simulink model "fusionAlg"  (R2018b)
settings: Solver=FixedStepDiscrete  StartTime=0.0  StopTime=inf  FixedStep=0.01  RelTol=1e-3
PostLoadFcn:
  | if any(exist('dsrtsu_mdlpostloadfcn', 'file') ~= 0), dsrtsu_mdlpostloadfcn('Execute', bdroot); end
model workspace (MAT data in the model file):
  handle : class17 (value not decoded)
(part 11 of 24)

== system fusionAlg/FUSION /FusionAlg/BusToBusArray/BusToBusArray/FUS_Obj_30 ==
  <fus_output_30_obj> : Inport
  Bus Creator : BusCreator  Inputs=15  OutDataTypeStr=Bus: FUS_OBJ_TRACK_EST_ST  NonVirtualBus=on
      settings: InheritFromInputs=off
  Bus Creator1 : BusCreator  Inputs=15  OutDataTypeStr=Bus: FUS_OBJ_TRACK_PROP_ST  NonVirtualBus=on
      settings: InheritFromInputs=off
  Bus Creator2 : BusCreator  Inputs=10  OutDataTypeStr=Bus: FUS_OBJ_TRACK_INFO_ST  NonVirtualBus=on
      settings: InheritFromInputs=off
  Bus Creator3 : BusCreator  Inputs=3  OutDataTypeStr=Bus: FUS_OBJ_DATA_ST  NonVirtualBus=on
      settings: InheritFromInputs=off
  Bus Selector : BusSelector  OutputSignals=obj_estimate,obj_property,obj_information
  Bus Selector1 : BusSelector  OutputSignals=longPosition,latPosition,headingAngle,speed,yawRate,longRelativeVelocity,latRelativeVelocity,longAbsoluteVelocity,latAbsoluteVelocity,acceleration,longRelativeAcceleration,latRelativeAcceleration,longAbsoluteAcceleration,latAbsoluteAcceleration,curvature
  Bus Selector2 : BusSelector  OutputSignals=id,fusionSource,motionModel,trackStatus,positionConfidence,fcwConfidence,tjaConfidence,leftNearLaneMarkingConfidence,rightNearLaneMarkingConfidence,visionId,accelerationStdDev,headingAngleStdDev,latPositionStdDev,longPositionStdDev,speedStdDev
  Bus Selector3 : BusSelector  OutputSignals=valid,type,nearestSide,motionPatternCurrent,motionPatternHistory,width,height,length,distanceToleftNearLaneMarking,distanceToRightNearLaneMarking
  BUS_fus_output_30_obj : Outport
  wires:
  <fus_output_30_obj>/1 -> Bus Selector/1
  Bus Selector/1 -> Bus Selector1/1  "<obj_estimate>"
  Bus Selector1/1 -> Bus Creator/1  "<longPosition>"
  Bus Selector1/2 -> Bus Creator/2  "<latPosition>"
  Bus Selector1/4 -> Bus Creator/4  "<speed>"
  Bus Selector1/5 -> Bus Creator/5  "<yawRate>"
  Bus Selector1/6 -> Bus Creator/6  "<longRelativeVelocity>"
  Bus Selector1/3 -> Bus Creator/3  "<headingAngle>"
  Bus Selector1/7 -> Bus Creator/7  "<latRelativeVelocity>"
  Bus Selector/2 -> Bus Selector2/1  "<obj_property>"
  Bus Selector/3 -> Bus Selector3/1  "<obj_information>"
  Bus Selector2/1 -> Bus Creator1/1  "<id>"
  Bus Selector2/2 -> Bus Creator1/2  "<fusionSource>"
  Bus Selector2/3 -> Bus Creator1/3  "<motionModel>"
  Bus Selector2/4 -> Bus Creator1/4  "<trackStatus>"
  Bus Selector2/6 -> Bus Creator1/6  "<fcwConfidence>"
  Bus Selector2/11 -> Bus Creator1/11  "<accelerationStdDev>"
  Bus Selector2/12 -> Bus Creator1/12  "<headingAngleStdDev>"
  Bus Selector2/13 -> Bus Creator1/13  "<latPositionStdDev>"
  Bus Selector2/14 -> Bus Creator1/14  "<longPositionStdDev>"
  Bus Selector2/15 -> Bus Creator1/15  "<speedStdDev>"
  Bus Selector2/9 -> Bus Creator1/9  "<rightNearLaneMarkingConfidence>"
  Bus Selector2/8 -> Bus Creator1/8  "<leftNearLaneMarkingConfidence>"
  Bus Selector2/10 -> Bus Creator1/10  "<visionId>"
  Bus Selector2/5 -> Bus Creator1/5  "<positionConfidence>"
  Bus Selector2/7 -> Bus Creator1/7  "<tjaConfidence>"
  Bus Selector3/1 -> Bus Creator2/1  "<valid>"
  Bus Selector3/2 -> Bus Creator2/2  "<type>"
  Bus Selector3/3 -> Bus Creator2/3  "<nearestSide>"
  Bus Selector3/4 -> Bus Creator2/4  "<motionPatternCurrent>"
  Bus Selector3/5 -> Bus Creator2/5  "<motionPatternHistory>"
  Bus Selector3/6 -> Bus Creator2/6  "<width>"
  Bus Selector3/7 -> Bus Creator2/7  "<height>"
  Bus Selector3/8 -> Bus Creator2/8  "<length>"
  Bus Selector3/9 -> Bus Creator2/9  "<distanceToleftNearLaneMarking>"
  Bus Creator/1 -> Bus Creator3/1
  Bus Creator1/1 -> Bus Creator3/2
  Bus Creator2/1 -> Bus Creator3/3
  Bus Creator3/1 -> BUS_fus_output_30_obj/1
  Bus Selector3/10 -> Bus Creator2/10  "<distanceToRightNearLaneMarking>"
  Bus Selector1/8 -> Bus Creator/8  "<longAbsoluteVelocity>"
  Bus Selector1/9 -> Bus Creator/9  "<latAbsoluteVelocity>"
  Bus Selector1/10 -> Bus Creator/10  "<acceleration>"
  Bus Selector1/11 -> Bus Creator/11  "<longRelativeAcceleration>"
  Bus Selector1/12 -> Bus Creator/12  "<latRelativeAcceleration>"
  Bus Selector1/13 -> Bus Creator/13  "<longAbsoluteAcceleration>"
  Bus Selector1/14 -> Bus Creator/14  "<latAbsoluteAcceleration>"
  Bus Selector1/15 -> Bus Creator/15  "<curvature>"

== system fusionAlg/FUSION /FusionAlg/BusToBusArray/BusToBusArray/FUS_Obj_31 ==
  <fus_output_31_obj> : Inport
  Bus Creator : BusCreator  Inputs=15  OutDataTypeStr=Bus: FUS_OBJ_TRACK_EST_ST  NonVirtualBus=on
      settings: InheritFromInputs=off
  Bus Creator1 : BusCreator  Inputs=15  OutDataTypeStr=Bus: FUS_OBJ_TRACK_PROP_ST  NonVirtualBus=on
      settings: InheritFromInputs=off
  Bus Creator2 : BusCreator  Inputs=10  OutDataTypeStr=Bus: FUS_OBJ_TRACK_INFO_ST  NonVirtualBus=on
      settings: InheritFromInputs=off
  Bus Creator3 : BusCreator  Inputs=3  OutDataTypeStr=Bus: FUS_OBJ_DATA_ST  NonVirtualBus=on
      settings: InheritFromInputs=off
  Bus Selector : BusSelector  OutputSignals=obj_estimate,obj_property,obj_information
  Bus Selector1 : BusSelector  OutputSignals=longPosition,latPosition,headingAngle,speed,yawRate,longRelativeVelocity,latRelativeVelocity,longAbsoluteVelocity,latAbsoluteVelocity,acceleration,longRelativeAcceleration,latRelativeAcceleration,longAbsoluteAcceleration,latAbsoluteAcceleration,curvature
  Bus Selector2 : BusSelector  OutputSignals=id,fusionSource,motionModel,trackStatus,positionConfidence,fcwConfidence,tjaConfidence,leftNearLaneMarkingConfidence,rightNearLaneMarkingConfidence,visionId,accelerationStdDev,headingAngleStdDev,latPositionStdDev,longPositionStdDev,speedStdDev
  Bus Selector3 : BusSelector  OutputSignals=valid,type,nearestSide,motionPatternCurrent,motionPatternHistory,width,height,length,distanceToleftNearLaneMarking,distanceToRightNearLaneMarking
  BUS_fus_output_31_obj : Outport
  wires:
  <fus_output_31_obj>/1 -> Bus Selector/1
  Bus Selector/1 -> Bus Selector1/1  "<obj_estimate>"
  Bus Selector1/1 -> Bus Creator/1  "<longPosition>"
  Bus Selector1/2 -> Bus Creator/2  "<latPosition>"
  Bus Selector1/4 -> Bus Creator/4  "<speed>"
  Bus Selector1/5 -> Bus Creator/5  "<yawRate>"
  Bus Selector1/6 -> Bus Creator/6  "<longRelativeVelocity>"
  Bus Selector1/3 -> Bus Creator/3  "<headingAngle>"
  Bus Selector1/7 -> Bus Creator/7  "<latRelativeVelocity>"
  Bus Selector/2 -> Bus Selector2/1  "<obj_property>"
  Bus Selector/3 -> Bus Selector3/1  "<obj_information>"
  Bus Selector2/1 -> Bus Creator1/1  "<id>"
  Bus Selector2/2 -> Bus Creator1/2  "<fusionSource>"
  Bus Selector2/3 -> Bus Creator1/3  "<motionModel>"
  Bus Selector2/4 -> Bus Creator1/4  "<trackStatus>"
  Bus Selector2/6 -> Bus Creator1/6  "<fcwConfidence>"
  Bus Selector2/11 -> Bus Creator1/11  "<accelerationStdDev>"
  Bus Selector2/12 -> Bus Creator1/12  "<headingAngleStdDev>"
  Bus Selector2/13 -> Bus Creator1/13  "<latPositionStdDev>"
  Bus Selector2/14 -> Bus Creator1/14  "<longPositionStdDev>"
  Bus Selector2/15 -> Bus Creator1/15  "<speedStdDev>"
  Bus Selector2/9 -> Bus Creator1/9  "<rightNearLaneMarkingConfidence>"
  Bus Selector2/8 -> Bus Creator1/8  "<leftNearLaneMarkingConfidence>"
  Bus Selector2/10 -> Bus Creator1/10  "<visionId>"
  Bus Selector2/5 -> Bus Creator1/5  "<positionConfidence>"
  Bus Selector2/7 -> Bus Creator1/7  "<tjaConfidence>"
  Bus Selector3/1 -> Bus Creator2/1  "<valid>"
  Bus Selector3/2 -> Bus Creator2/2  "<type>"
  Bus Selector3/3 -> Bus Creator2/3  "<nearestSide>"
  Bus Selector3/4 -> Bus Creator2/4  "<motionPatternCurrent>"
  Bus Selector3/5 -> Bus Creator2/5  "<motionPatternHistory>"
  Bus Selector3/6 -> Bus Creator2/6  "<width>"
  Bus Selector3/7 -> Bus Creator2/7  "<height>"
  Bus Selector3/8 -> Bus Creator2/8  "<length>"
  Bus Selector3/9 -> Bus Creator2/9  "<distanceToleftNearLaneMarking>"
  Bus Creator/1 -> Bus Creator3/1
  Bus Creator1/1 -> Bus Creator3/2
  Bus Creator2/1 -> Bus Creator3/3
  Bus Creator3/1 -> BUS_fus_output_31_obj/1
  Bus Selector3/10 -> Bus Creator2/10  "<distanceToRightNearLaneMarking>"
  Bus Selector1/8 -> Bus Creator/8  "<longAbsoluteVelocity>"
  Bus Selector1/9 -> Bus Creator/9  "<latAbsoluteVelocity>"
  Bus Selector1/10 -> Bus Creator/10  "<acceleration>"
  Bus Selector1/11 -> Bus Creator/11  "<longRelativeAcceleration>"
  Bus Selector1/12 -> Bus Creator/12  "<latRelativeAcceleration>"
  Bus Selector1/13 -> Bus Creator/13  "<longAbsoluteAcceleration>"
  Bus Selector1/14 -> Bus Creator/14  "<latAbsoluteAcceleration>"
  Bus Selector1/15 -> Bus Creator/15  "<curvature>"

== system fusionAlg/FUSION /FusionAlg/BusToBusArray/BusToBusArray/FUS_Obj_32 ==
  <fus_output_32_obj> : Inport
  Bus Creator : BusCreator  Inputs=15  OutDataTypeStr=Bus: FUS_OBJ_TRACK_EST_ST  NonVirtualBus=on
      settings: InheritFromInputs=off
  Bus Creator1 : BusCreator  Inputs=15  OutDataTypeStr=Bus: FUS_OBJ_TRACK_PROP_ST  NonVirtualBus=on
      settings: InheritFromInputs=off
  Bus Creator2 : BusCreator  Inputs=10  OutDataTypeStr=Bus: FUS_OBJ_TRACK_INFO_ST  NonVirtualBus=on
      settings: InheritFromInputs=off
  Bus Creator3 : BusCreator  Inputs=3  OutDataTypeStr=Bus: FUS_OBJ_DATA_ST  NonVirtualBus=on
      settings: InheritFromInputs=off
  Bus Selector : BusSelector  OutputSignals=obj_estimate,obj_property,obj_information
  Bus Selector1 : BusSelector  OutputSignals=longPosition,latPosition,headingAngle,speed,yawRate,longRelativeVelocity,latRelativeVelocity,longAbsoluteVelocity,latAbsoluteVelocity,acceleration,longRelativeAcceleration,latRelativeAcceleration,longAbsoluteAcceleration,latAbsoluteAcceleration,curvature
  Bus Selector2 : BusSelector  OutputSignals=id,fusionSource,motionModel,trackStatus,positionConfidence,fcwConfidence,tjaConfidence,leftNearLaneMarkingConfidence,rightNearLaneMarkingConfidence,visionId,accelerationStdDev,headingAngleStdDev,latPositionStdDev,longPositionStdDev,speedStdDev
  Bus Selector3 : BusSelector  OutputSignals=valid,type,nearestSide,motionPatternCurrent,motionPatternHistory,width,height,length,distanceToleftNearLaneMarking,distanceToRightNearLaneMarking
  BUS_fus_output_32_obj : Outport
  wires:
  <fus_output_32_obj>/1 -> Bus Selector/1
  Bus Selector/1 -> Bus Selector1/1  "<obj_estimate>"
  Bus Selector1/1 -> Bus Creator/1  "<longPosition>"
  Bus Selector1/2 -> Bus Creator/2  "<latPosition>"
  Bus Selector1/4 -> Bus Creator/4  "<speed>"
  Bus Selector1/5 -> Bus Creator/5  "<yawRate>"
  Bus Selector1/6 -> Bus Creator/6  "<longRelativeVelocity>"
  Bus Selector1/3 -> Bus Creator/3  "<headingAngle>"
  Bus Selector1/7 -> Bus Creator/7  "<latRelativeVelocity>"
  Bus Selector/2 -> Bus Selector2/1  "<obj_property>"
  Bus Selector/3 -> Bus Selector3/1  "<obj_information>"
  Bus Selector2/1 -> Bus Creator1/1  "<id>"
  Bus Selector2/2 -> Bus Creator1/2  "<fusionSource>"
  Bus Selector2/3 -> Bus Creator1/3  "<motionModel>"
  Bus Selector2/4 -> Bus Creator1/4  "<trackStatus>"
  Bus Selector2/6 -> Bus Creator1/6  "<fcwConfidence>"
  Bus Selector2/11 -> Bus Creator1/11  "<accelerationStdDev>"
  Bus Selector2/12 -> Bus Creator1/12  "<headingAngleStdDev>"
  Bus Selector2/13 -> Bus Creator1/13  "<latPositionStdDev>"
  Bus Selector2/14 -> Bus Creator1/14  "<longPositionStdDev>"
  Bus Selector2/15 -> Bus Creator1/15  "<speedStdDev>"
  Bus Selector2/9 -> Bus Creator1/9  "<rightNearLaneMarkingConfidence>"
  Bus Selector2/8 -> Bus Creator1/8  "<leftNearLaneMarkingConfidence>"
  Bus Selector2/10 -> Bus Creator1/10  "<visionId>"
  Bus Selector2/5 -> Bus Creator1/5  "<positionConfidence>"
  Bus Selector2/7 -> Bus Creator1/7  "<tjaConfidence>"
  Bus Selector3/1 -> Bus Creator2/1  "<valid>"
  Bus Selector3/2 -> Bus Creator2/2  "<type>"
  Bus Selector3/3 -> Bus Creator2/3  "<nearestSide>"
  Bus Selector3/4 -> Bus Creator2/4  "<motionPatternCurrent>"
  Bus Selector3/5 -> Bus Creator2/5  "<motionPatternHistory>"
  Bus Selector3/6 -> Bus Creator2/6  "<width>"
  Bus Selector3/7 -> Bus Creator2/7  "<height>"
  Bus Selector3/8 -> Bus Creator2/8  "<length>"
  Bus Selector3/9 -> Bus Creator2/9  "<distanceToleftNearLaneMarking>"
  Bus Creator/1 -> Bus Creator3/1
  Bus Creator1/1 -> Bus Creator3/2
  Bus Creator2/1 -> Bus Creator3/3
  Bus Creator3/1 -> BUS_fus_output_32_obj/1
  Bus Selector3/10 -> Bus Creator2/10  "<distanceToRightNearLaneMarking>"
  Bus Selector1/8 -> Bus Creator/8  "<longAbsoluteVelocity>"
  Bus Selector1/9 -> Bus Creator/9  "<latAbsoluteVelocity>"
  Bus Selector1/10 -> Bus Creator/10  "<acceleration>"
  Bus Selector1/11 -> Bus Creator/11  "<longRelativeAcceleration>"
  Bus Selector1/12 -> Bus Creator/12  "<latRelativeAcceleration>"
  Bus Selector1/13 -> Bus Creator/13  "<longAbsoluteAcceleration>"
  Bus Selector1/14 -> Bus Creator/14  "<latAbsoluteAcceleration>"
  Bus Selector1/15 -> Bus Creator/15  "<curvature>"

== system fusionAlg/FUSION /FusionAlg/BusToBusArray/BusToBusArray/FUS_Obj_33 ==
  <fus_output_33_obj> : Inport
  Bus Creator : BusCreator  Inputs=15  OutDataTypeStr=Bus: FUS_OBJ_TRACK_EST_ST  NonVirtualBus=on
      settings: InheritFromInputs=off
  Bus Creator1 : BusCreator  Inputs=15  OutDataTypeStr=Bus: FUS_OBJ_TRACK_PROP_ST  NonVirtualBus=on
      settings: InheritFromInputs=off
  Bus Creator2 : BusCreator  Inputs=10  OutDataTypeStr=Bus: FUS_OBJ_TRACK_INFO_ST  NonVirtualBus=on
      settings: InheritFromInputs=off
  Bus Creator3 : BusCreator  Inputs=3  OutDataTypeStr=Bus: FUS_OBJ_DATA_ST  NonVirtualBus=on
      settings: InheritFromInputs=off
  Bus Selector : BusSelector  OutputSignals=obj_estimate,obj_property,obj_information
  Bus Selector1 : BusSelector  OutputSignals=longPosition,latPosition,headingAngle,speed,yawRate,longRelativeVelocity,latRelativeVelocity,longAbsoluteVelocity,latAbsoluteVelocity,acceleration,longRelativeAcceleration,latRelativeAcceleration,longAbsoluteAcceleration,latAbsoluteAcceleration,curvature
  Bus Selector2 : BusSelector  OutputSignals=id,fusionSource,motionModel,trackStatus,positionConfidence,fcwConfidence,tjaConfidence,leftNearLaneMarkingConfidence,rightNearLaneMarkingConfidence,visionId,accelerationStdDev,headingAngleStdDev,latPositionStdDev,longPositionStdDev,speedStdDev
  Bus Selector3 : BusSelector  OutputSignals=valid,type,nearestSide,motionPatternCurrent,motionPatternHistory,width,height,length,distanceToleftNearLaneMarking,distanceToRightNearLaneMarking
  BUS_fus_output_33_obj : Outport
  wires:
  <fus_output_33_obj>/1 -> Bus Selector/1
  Bus Selector/1 -> Bus Selector1/1  "<obj_estimate>"
  Bus Selector1/1 -> Bus Creator/1  "<longPosition>"
  Bus Selector1/2 -> Bus Creator/2  "<latPosition>"
  Bus Selector1/4 -> Bus Creator/4  "<speed>"
  Bus Selector1/5 -> Bus Creator/5  "<yawRate>"
  Bus Selector1/6 -> Bus Creator/6  "<longRelativeVelocity>"
  Bus Selector1/3 -> Bus Creator/3  "<headingAngle>"
  Bus Selector1/7 -> Bus Creator/7  "<latRelativeVelocity>"
  Bus Selector/2 -> Bus Selector2/1  "<obj_property>"
  Bus Selector/3 -> Bus Selector3/1  "<obj_information>"
  Bus Selector2/1 -> Bus Creator1/1  "<id>"
  Bus Selector2/2 -> Bus Creator1/2  "<fusionSource>"
  Bus Selector2/3 -> Bus Creator1/3  "<motionModel>"
  Bus Selector2/4 -> Bus Creator1/4  "<trackStatus>"
  Bus Selector2/6 -> Bus Creator1/6  "<fcwConfidence>"
  Bus Selector2/11 -> Bus Creator1/11  "<accelerationStdDev>"
  Bus Selector2/12 -> Bus Creator1/12  "<headingAngleStdDev>"
  Bus Selector2/13 -> Bus Creator1/13  "<latPositionStdDev>"
  Bus Selector2/14 -> Bus Creator1/14  "<longPositionStdDev>"
  Bus Selector2/15 -> Bus Creator1/15  "<speedStdDev>"
  Bus Selector2/9 -> Bus Creator1/9  "<rightNearLaneMarkingConfidence>"
  Bus Selector2/8 -> Bus Creator1/8  "<leftNearLaneMarkingConfidence>"
  Bus Selector2/10 -> Bus Creator1/10  "<visionId>"
  Bus Selector2/5 -> Bus Creator1/5  "<positionConfidence>"
  Bus Selector2/7 -> Bus Creator1/7  "<tjaConfidence>"
  Bus Selector3/1 -> Bus Creator2/1  "<valid>"
  Bus Selector3/2 -> Bus Creator2/2  "<type>"
  Bus Selector3/3 -> Bus Creator2/3  "<nearestSide>"
  Bus Selector3/4 -> Bus Creator2/4  "<motionPatternCurrent>"
  Bus Selector3/5 -> Bus Creator2/5  "<motionPatternHistory>"
  Bus Selector3/6 -> Bus Creator2/6  "<width>"
  Bus Selector3/7 -> Bus Creator2/7  "<height>"
  Bus Selector3/8 -> Bus Creator2/8  "<length>"
  Bus Selector3/9 -> Bus Creator2/9  "<distanceToleftNearLaneMarking>"
  Bus Creator/1 -> Bus Creator3/1
  Bus Creator1/1 -> Bus Creator3/2
  Bus Creator2/1 -> Bus Creator3/3
  Bus Creator3/1 -> BUS_fus_output_33_obj/1
  Bus Selector3/10 -> Bus Creator2/10  "<distanceToRightNearLaneMarking>"
  Bus Selector1/8 -> Bus Creator/8  "<longAbsoluteVelocity>"
  Bus Selector1/9 -> Bus Creator/9  "<latAbsoluteVelocity>"
  Bus Selector1/10 -> Bus Creator/10  "<acceleration>"
  Bus Selector1/11 -> Bus Creator/11  "<longRelativeAcceleration>"
  Bus Selector1/12 -> Bus Creator/12  "<latRelativeAcceleration>"
  Bus Selector1/13 -> Bus Creator/13  "<longAbsoluteAcceleration>"
  Bus Selector1/14 -> Bus Creator/14  "<latAbsoluteAcceleration>"
  Bus Selector1/15 -> Bus Creator/15  "<curvature>"

== system fusionAlg/FUSION /FusionAlg/BusToBusArray/BusToBusArray/FUS_Obj_34 ==
  <fus_output_34_obj> : Inport
  Bus Creator : BusCreator  Inputs=15  OutDataTypeStr=Bus: FUS_OBJ_TRACK_EST_ST  NonVirtualBus=on
      settings: InheritFromInputs=off
  Bus Creator1 : BusCreator  Inputs=15  OutDataTypeStr=Bus: FUS_OBJ_TRACK_PROP_ST  NonVirtualBus=on
      settings: InheritFromInputs=off
  Bus Creator2 : BusCreator  Inputs=10  OutDataTypeStr=Bus: FUS_OBJ_TRACK_INFO_ST  NonVirtualBus=on
      settings: InheritFromInputs=off
  Bus Creator3 : BusCreator  Inputs=3  OutDataTypeStr=Bus: FUS_OBJ_DATA_ST  NonVirtualBus=on
      settings: InheritFromInputs=off
  Bus Selector : BusSelector  OutputSignals=obj_estimate,obj_property,obj_information
  Bus Selector1 : BusSelector  OutputSignals=longPosition,latPosition,headingAngle,speed,yawRate,longRelativeVelocity,latRelativeVelocity,longAbsoluteVelocity,latAbsoluteVelocity,acceleration,longRelativeAcceleration,latRelativeAcceleration,longAbsoluteAcceleration,latAbsoluteAcceleration,curvature
  Bus Selector2 : BusSelector  OutputSignals=id,fusionSource,motionModel,trackStatus,positionConfidence,fcwConfidence,tjaConfidence,leftNearLaneMarkingConfidence,rightNearLaneMarkingConfidence,visionId,accelerationStdDev,headingAngleStdDev,latPositionStdDev,longPositionStdDev,speedStdDev
  Bus Selector3 : BusSelector  OutputSignals=valid,type,nearestSide,motionPatternCurrent,motionPatternHistory,width,height,length,distanceToleftNearLaneMarking,distanceToRightNearLaneMarking
  BUS_fus_output_34_obj : Outport
  wires:
  <fus_output_34_obj>/1 -> Bus Selector/1
  Bus Selector/1 -> Bus Selector1/1  "<obj_estimate>"
  Bus Selector1/1 -> Bus Creator/1  "<longPosition>"
  Bus Selector1/2 -> Bus Creator/2  "<latPosition>"
  Bus Selector1/4 -> Bus Creator/4  "<speed>"
  Bus Selector1/5 -> Bus Creator/5  "<yawRate>"
  Bus Selector1/6 -> Bus Creator/6  "<longRelativeVelocity>"
  Bus Selector1/3 -> Bus Creator/3  "<headingAngle>"
  Bus Selector1/7 -> Bus Creator/7  "<latRelativeVelocity>"
  Bus Selector/2 -> Bus Selector2/1  "<obj_property>"
  Bus Selector/3 -> Bus Selector3/1  "<obj_information>"
  Bus Selector2/1 -> Bus Creator1/1  "<id>"
  Bus Selector2/2 -> Bus Creator1/2  "<fusionSource>"
  Bus Selector2/3 -> Bus Creator1/3  "<motionModel>"
  Bus Selector2/4 -> Bus Creator1/4  "<trackStatus>"
  Bus Selector2/6 -> Bus Creator1/6  "<fcwConfidence>"
  Bus Selector2/11 -> Bus Creator1/11  "<accelerationStdDev>"
  Bus Selector2/12 -> Bus Creator1/12  "<headingAngleStdDev>"
  Bus Selector2/13 -> Bus Creator1/13  "<latPositionStdDev>"
  Bus Selector2/14 -> Bus Creator1/14  "<longPositionStdDev>"
  Bus Selector2/15 -> Bus Creator1/15  "<speedStdDev>"
  Bus Selector2/9 -> Bus Creator1/9  "<rightNearLaneMarkingConfidence>"
  Bus Selector2/8 -> Bus Creator1/8  "<leftNearLaneMarkingConfidence>"
  Bus Selector2/10 -> Bus Creator1/10  "<visionId>"
  Bus Selector2/5 -> Bus Creator1/5  "<positionConfidence>"
  Bus Selector2/7 -> Bus Creator1/7  "<tjaConfidence>"
  Bus Selector3/1 -> Bus Creator2/1  "<valid>"
  Bus Selector3/2 -> Bus Creator2/2  "<type>"
  Bus Selector3/3 -> Bus Creator2/3  "<nearestSide>"
  Bus Selector3/4 -> Bus Creator2/4  "<motionPatternCurrent>"
  Bus Selector3/5 -> Bus Creator2/5  "<motionPatternHistory>"
  Bus Selector3/6 -> Bus Creator2/6  "<width>"
  Bus Selector3/7 -> Bus Creator2/7  "<height>"
  Bus Selector3/8 -> Bus Creator2/8  "<length>"
  Bus Selector3/9 -> Bus Creator2/9  "<distanceToleftNearLaneMarking>"
  Bus Creator/1 -> Bus Creator3/1
  Bus Creator1/1 -> Bus Creator3/2
  Bus Creator2/1 -> Bus Creator3/3
  Bus Creator3/1 -> BUS_fus_output_34_obj/1
  Bus Selector3/10 -> Bus Creator2/10  "<distanceToRightNearLaneMarking>"
  Bus Selector1/8 -> Bus Creator/8  "<longAbsoluteVelocity>"
  Bus Selector1/9 -> Bus Creator/9  "<latAbsoluteVelocity>"
  Bus Selector1/10 -> Bus Creator/10  "<acceleration>"
  Bus Selector1/11 -> Bus Creator/11  "<longRelativeAcceleration>"
  Bus Selector1/12 -> Bus Creator/12  "<latRelativeAcceleration>"
  Bus Selector1/13 -> Bus Creator/13  "<longAbsoluteAcceleration>"
  Bus Selector1/14 -> Bus Creator/14  "<latAbsoluteAcceleration>"
  Bus Selector1/15 -> Bus Creator/15  "<curvature>"

== system fusionAlg/FUSION /FusionAlg/BusToBusArray/BusToBusArray/FUS_Obj_35 ==
  <fus_output_35_obj> : Inport
  Bus Creator : BusCreator  Inputs=15  OutDataTypeStr=Bus: FUS_OBJ_TRACK_EST_ST  NonVirtualBus=on
      settings: InheritFromInputs=off
  Bus Creator1 : BusCreator  Inputs=15  OutDataTypeStr=Bus: FUS_OBJ_TRACK_PROP_ST  NonVirtualBus=on
      settings: InheritFromInputs=off
  Bus Creator2 : BusCreator  Inputs=10  OutDataTypeStr=Bus: FUS_OBJ_TRACK_INFO_ST  NonVirtualBus=on
      settings: InheritFromInputs=off
  Bus Creator3 : BusCreator  Inputs=3  OutDataTypeStr=Bus: FUS_OBJ_DATA_ST  NonVirtualBus=on
      settings: InheritFromInputs=off
  Bus Selector : BusSelector  OutputSignals=obj_estimate,obj_property,obj_information
  Bus Selector1 : BusSelector  OutputSignals=longPosition,latPosition,headingAngle,speed,yawRate,longRelativeVelocity,latRelativeVelocity,longAbsoluteVelocity,latAbsoluteVelocity,acceleration,longRelativeAcceleration,latRelativeAcceleration,longAbsoluteAcceleration,latAbsoluteAcceleration,curvature
  Bus Selector2 : BusSelector  OutputSignals=id,fusionSource,motionModel,trackStatus,positionConfidence,fcwConfidence,tjaConfidence,leftNearLaneMarkingConfidence,rightNearLaneMarkingConfidence,visionId,accelerationStdDev,headingAngleStdDev,latPositionStdDev,longPositionStdDev,speedStdDev
  Bus Selector3 : BusSelector  OutputSignals=valid,type,nearestSide,motionPatternCurrent,motionPatternHistory,width,height,length,distanceToleftNearLaneMarking,distanceToRightNearLaneMarking
  BUS_fus_output_35_obj : Outport
  wires:
  <fus_output_35_obj>/1 -> Bus Selector/1
  Bus Selector/1 -> Bus Selector1/1  "<obj_estimate>"
  Bus Selector1/1 -> Bus Creator/1  "<longPosition>"
  Bus Selector1/2 -> Bus Creator/2  "<latPosition>"
  Bus Selector1/4 -> Bus Creator/4  "<speed>"
  Bus Selector1/5 -> Bus Creator/5  "<yawRate>"
  Bus Selector1/6 -> Bus Creator/6  "<longRelativeVelocity>"
  Bus Selector1/3 -> Bus Creator/3  "<headingAngle>"
  Bus Selector1/7 -> Bus Creator/7  "<latRelativeVelocity>"
  Bus Selector/2 -> Bus Selector2/1  "<obj_property>"
  Bus Selector/3 -> Bus Selector3/1  "<obj_information>"
  Bus Selector2/1 -> Bus Creator1/1  "<id>"
  Bus Selector2/2 -> Bus Creator1/2  "<fusionSource>"
  Bus Selector2/3 -> Bus Creator1/3  "<motionModel>"
  Bus Selector2/4 -> Bus Creator1/4  "<trackStatus>"
  Bus Selector2/6 -> Bus Creator1/6  "<fcwConfidence>"
  Bus Selector2/11 -> Bus Creator1/11  "<accelerationStdDev>"
  Bus Selector2/12 -> Bus Creator1/12  "<headingAngleStdDev>"
  Bus Selector2/13 -> Bus Creator1/13  "<latPositionStdDev>"
  Bus Selector2/14 -> Bus Creator1/14  "<longPositionStdDev>"
  Bus Selector2/15 -> Bus Creator1/15  "<speedStdDev>"
  Bus Selector2/9 -> Bus Creator1/9  "<rightNearLaneMarkingConfidence>"
  Bus Selector2/8 -> Bus Creator1/8  "<leftNearLaneMarkingConfidence>"
  Bus Selector2/10 -> Bus Creator1/10  "<visionId>"
  Bus Selector2/5 -> Bus Creator1/5  "<positionConfidence>"
  Bus Selector2/7 -> Bus Creator1/7  "<tjaConfidence>"
  Bus Selector3/1 -> Bus Creator2/1  "<valid>"
  Bus Selector3/2 -> Bus Creator2/2  "<type>"
  Bus Selector3/3 -> Bus Creator2/3  "<nearestSide>"
  Bus Selector3/4 -> Bus Creator2/4  "<motionPatternCurrent>"
  Bus Selector3/5 -> Bus Creator2/5  "<motionPatternHistory>"
  Bus Selector3/6 -> Bus Creator2/6  "<width>"
  Bus Selector3/7 -> Bus Creator2/7  "<height>"
  Bus Selector3/8 -> Bus Creator2/8  "<length>"
  Bus Selector3/9 -> Bus Creator2/9  "<distanceToleftNearLaneMarking>"
  Bus Creator/1 -> Bus Creator3/1
  Bus Creator1/1 -> Bus Creator3/2
  Bus Creator2/1 -> Bus Creator3/3
  Bus Creator3/1 -> BUS_fus_output_35_obj/1
  Bus Selector3/10 -> Bus Creator2/10  "<distanceToRightNearLaneMarking>"
  Bus Selector1/8 -> Bus Creator/8  "<longAbsoluteVelocity>"
  Bus Selector1/9 -> Bus Creator/9  "<latAbsoluteVelocity>"
  Bus Selector1/10 -> Bus Creator/10  "<acceleration>"
  Bus Selector1/11 -> Bus Creator/11  "<longRelativeAcceleration>"
  Bus Selector1/12 -> Bus Creator/12  "<latRelativeAcceleration>"
  Bus Selector1/13 -> Bus Creator/13  "<longAbsoluteAcceleration>"
  Bus Selector1/14 -> Bus Creator/14  "<latAbsoluteAcceleration>"
  Bus Selector1/15 -> Bus Creator/15  "<curvature>"

== system fusionAlg/FUSION /FusionAlg/BusToBusArray/BusToBusArray/FUS_Obj_36 ==
  <fus_output_36_obj> : Inport
  Bus Creator : BusCreator  Inputs=15  OutDataTypeStr=Bus: FUS_OBJ_TRACK_EST_ST  NonVirtualBus=on
      settings: InheritFromInputs=off
  Bus Creator1 : BusCreator  Inputs=15  OutDataTypeStr=Bus: FUS_OBJ_TRACK_PROP_ST  NonVirtualBus=on
      settings: InheritFromInputs=off
  Bus Creator2 : BusCreator  Inputs=10  OutDataTypeStr=Bus: FUS_OBJ_TRACK_INFO_ST  NonVirtualBus=on
      settings: InheritFromInputs=off
  Bus Creator3 : BusCreator  Inputs=3  OutDataTypeStr=Bus: FUS_OBJ_DATA_ST  NonVirtualBus=on
      settings: InheritFromInputs=off
  Bus Selector : BusSelector  OutputSignals=obj_estimate,obj_property,obj_information
  Bus Selector1 : BusSelector  OutputSignals=longPosition,latPosition,headingAngle,speed,yawRate,longRelativeVelocity,latRelativeVelocity,longAbsoluteVelocity,latAbsoluteVelocity,acceleration,longRelativeAcceleration,latRelativeAcceleration,longAbsoluteAcceleration,latAbsoluteAcceleration,curvature
  Bus Selector2 : BusSelector  OutputSignals=id,fusionSource,motionModel,trackStatus,positionConfidence,fcwConfidence,tjaConfidence,leftNearLaneMarkingConfidence,rightNearLaneMarkingConfidence,visionId,accelerationStdDev,headingAngleStdDev,latPositionStdDev,longPositionStdDev,speedStdDev
  Bus Selector3 : BusSelector  OutputSignals=valid,type,nearestSide,motionPatternCurrent,motionPatternHistory,width,height,length,distanceToleftNearLaneMarking,distanceToRightNearLaneMarking
  BUS_fus_output_36_obj : Outport
  wires:
  <fus_output_36_obj>/1 -> Bus Selector/1
  Bus Selector/1 -> Bus Selector1/1  "<obj_estimate>"
  Bus Selector1/1 -> Bus Creator/1  "<longPosition>"
  Bus Selector1/2 -> Bus Creator/2  "<latPosition>"
  Bus Selector1/4 -> Bus Creator/4  "<speed>"
  Bus Selector1/5 -> Bus Creator/5  "<yawRate>"
  Bus Selector1/6 -> Bus Creator/6  "<longRelativeVelocity>"
  Bus Selector1/3 -> Bus Creator/3  "<headingAngle>"
  Bus Selector1/7 -> Bus Creator/7  "<latRelativeVelocity>"
  Bus Selector/2 -> Bus Selector2/1  "<obj_property>"
  Bus Selector/3 -> Bus Selector3/1  "<obj_information>"
  Bus Selector2/1 -> Bus Creator1/1  "<id>"
  Bus Selector2/2 -> Bus Creator1/2  "<fusionSource>"
  Bus Selector2/3 -> Bus Creator1/3  "<motionModel>"
  Bus Selector2/4 -> Bus Creator1/4  "<trackStatus>"
  Bus Selector2/6 -> Bus Creator1/6  "<fcwConfidence>"
  Bus Selector2/11 -> Bus Creator1/11  "<accelerationStdDev>"
  Bus Selector2/12 -> Bus Creator1/12  "<headingAngleStdDev>"
  Bus Selector2/13 -> Bus Creator1/13  "<latPositionStdDev>"
  Bus Selector2/14 -> Bus Creator1/14  "<longPositionStdDev>"
  Bus Selector2/15 -> Bus Creator1/15  "<speedStdDev>"
  Bus Selector2/9 -> Bus Creator1/9  "<rightNearLaneMarkingConfidence>"
  Bus Selector2/8 -> Bus Creator1/8  "<leftNearLaneMarkingConfidence>"
  Bus Selector2/10 -> Bus Creator1/10  "<visionId>"
  Bus Selector2/5 -> Bus Creator1/5  "<positionConfidence>"
  Bus Selector2/7 -> Bus Creator1/7  "<tjaConfidence>"
  Bus Selector3/1 -> Bus Creator2/1  "<valid>"
  Bus Selector3/2 -> Bus Creator2/2  "<type>"
  Bus Selector3/3 -> Bus Creator2/3  "<nearestSide>"
  Bus Selector3/4 -> Bus Creator2/4  "<motionPatternCurrent>"
  Bus Selector3/5 -> Bus Creator2/5  "<motionPatternHistory>"
  Bus Selector3/6 -> Bus Creator2/6  "<width>"
  Bus Selector3/7 -> Bus Creator2/7  "<height>"
  Bus Selector3/8 -> Bus Creator2/8  "<length>"
  Bus Selector3/9 -> Bus Creator2/9  "<distanceToleftNearLaneMarking>"
  Bus Creator/1 -> Bus Creator3/1
  Bus Creator1/1 -> Bus Creator3/2
  Bus Creator2/1 -> Bus Creator3/3
  Bus Creator3/1 -> BUS_fus_output_36_obj/1
  Bus Selector3/10 -> Bus Creator2/10  "<distanceToRightNearLaneMarking>"
  Bus Selector1/8 -> Bus Creator/8  "<longAbsoluteVelocity>"
  Bus Selector1/9 -> Bus Creator/9  "<latAbsoluteVelocity>"
  Bus Selector1/10 -> Bus Creator/10  "<acceleration>"
  Bus Selector1/11 -> Bus Creator/11  "<longRelativeAcceleration>"
  Bus Selector1/12 -> Bus Creator/12  "<latRelativeAcceleration>"
  Bus Selector1/13 -> Bus Creator/13  "<longAbsoluteAcceleration>"
  Bus Selector1/14 -> Bus Creator/14  "<latAbsoluteAcceleration>"
  Bus Selector1/15 -> Bus Creator/15  "<curvature>"

== system fusionAlg/FUSION /FusionAlg/BusToBusArray/BusToBusArray/FUS_Obj_37 ==
  <fus_output_37_obj> : Inport
  Bus Creator : BusCreator  Inputs=15  OutDataTypeStr=Bus: FUS_OBJ_TRACK_EST_ST  NonVirtualBus=on
      settings: InheritFromInputs=off
  Bus Creator1 : BusCreator  Inputs=15  OutDataTypeStr=Bus: FUS_OBJ_TRACK_PROP_ST  NonVirtualBus=on
      settings: InheritFromInputs=off
  Bus Creator2 : BusCreator  Inputs=10  OutDataTypeStr=Bus: FUS_OBJ_TRACK_INFO_ST  NonVirtualBus=on
      settings: InheritFromInputs=off
  Bus Creator3 : BusCreator  Inputs=3  OutDataTypeStr=Bus: FUS_OBJ_DATA_ST  NonVirtualBus=on
      settings: InheritFromInputs=off
  Bus Selector : BusSelector  OutputSignals=obj_estimate,obj_property,obj_information
  Bus Selector1 : BusSelector  OutputSignals=longPosition,latPosition,headingAngle,speed,yawRate,longRelativeVelocity,latRelativeVelocity,longAbsoluteVelocity,latAbsoluteVelocity,acceleration,longRelativeAcceleration,latRelativeAcceleration,longAbsoluteAcceleration,latAbsoluteAcceleration,curvature
  Bus Selector2 : BusSelector  OutputSignals=id,fusionSource,motionModel,trackStatus,positionConfidence,fcwConfidence,tjaConfidence,leftNearLaneMarkingConfidence,rightNearLaneMarkingConfidence,visionId,accelerationStdDev,headingAngleStdDev,latPositionStdDev,longPositionStdDev,speedStdDev
  Bus Selector3 : BusSelector  OutputSignals=valid,type,nearestSide,motionPatternCurrent,motionPatternHistory,width,height,length,distanceToleftNearLaneMarking,distanceToRightNearLaneMarking
  BUS_fus_output_37_obj : Outport
  wires:
  <fus_output_37_obj>/1 -> Bus Selector/1
  Bus Selector/1 -> Bus Selector1/1  "<obj_estimate>"
  Bus Selector1/1 -> Bus Creator/1  "<longPosition>"
  Bus Selector1/2 -> Bus Creator/2  "<latPosition>"
  Bus Selector1/4 -> Bus Creator/4  "<speed>"
  Bus Selector1/5 -> Bus Creator/5  "<yawRate>"
  Bus Selector1/6 -> Bus Creator/6  "<longRelativeVelocity>"
  Bus Selector1/3 -> Bus Creator/3  "<headingAngle>"
  Bus Selector1/7 -> Bus Creator/7  "<latRelativeVelocity>"
  Bus Selector/2 -> Bus Selector2/1  "<obj_property>"
  Bus Selector/3 -> Bus Selector3/1  "<obj_information>"
  Bus Selector2/1 -> Bus Creator1/1  "<id>"
  Bus Selector2/2 -> Bus Creator1/2  "<fusionSource>"
  Bus Selector2/3 -> Bus Creator1/3  "<motionModel>"
  Bus Selector2/4 -> Bus Creator1/4  "<trackStatus>"
  Bus Selector2/6 -> Bus Creator1/6  "<fcwConfidence>"
  Bus Selector2/11 -> Bus Creator1/11  "<accelerationStdDev>"
  Bus Selector2/12 -> Bus Creator1/12  "<headingAngleStdDev>"
  Bus Selector2/13 -> Bus Creator1/13  "<latPositionStdDev>"
  Bus Selector2/14 -> Bus Creator1/14  "<longPositionStdDev>"
  Bus Selector2/15 -> Bus Creator1/15  "<speedStdDev>"
  Bus Selector2/9 -> Bus Creator1/9  "<rightNearLaneMarkingConfidence>"
  Bus Selector2/8 -> Bus Creator1/8  "<leftNearLaneMarkingConfidence>"
  Bus Selector2/10 -> Bus Creator1/10  "<visionId>"
  Bus Selector2/5 -> Bus Creator1/5  "<positionConfidence>"
  Bus Selector2/7 -> Bus Creator1/7  "<tjaConfidence>"
  Bus Selector3/1 -> Bus Creator2/1  "<valid>"
  Bus Selector3/2 -> Bus Creator2/2  "<type>"
  Bus Selector3/3 -> Bus Creator2/3  "<nearestSide>"
  Bus Selector3/4 -> Bus Creator2/4  "<motionPatternCurrent>"
  Bus Selector3/5 -> Bus Creator2/5  "<motionPatternHistory>"
  Bus Selector3/6 -> Bus Creator2/6  "<width>"
  Bus Selector3/7 -> Bus Creator2/7  "<height>"
  Bus Selector3/8 -> Bus Creator2/8  "<length>"
  Bus Selector3/9 -> Bus Creator2/9  "<distanceToleftNearLaneMarking>"
  Bus Creator/1 -> Bus Creator3/1
  Bus Creator1/1 -> Bus Creator3/2
  Bus Creator2/1 -> Bus Creator3/3
  Bus Creator3/1 -> BUS_fus_output_37_obj/1
  Bus Selector3/10 -> Bus Creator2/10  "<distanceToRightNearLaneMarking>"
  Bus Selector1/8 -> Bus Creator/8  "<longAbsoluteVelocity>"
  Bus Selector1/9 -> Bus Creator/9  "<latAbsoluteVelocity>"
  Bus Selector1/10 -> Bus Creator/10  "<acceleration>"
  Bus Selector1/11 -> Bus Creator/11  "<longRelativeAcceleration>"
  Bus Selector1/12 -> Bus Creator/12  "<latRelativeAcceleration>"
  Bus Selector1/13 -> Bus Creator/13  "<longAbsoluteAcceleration>"
  Bus Selector1/14 -> Bus Creator/14  "<latAbsoluteAcceleration>"
  Bus Selector1/15 -> Bus Creator/15  "<curvature>"

== system fusionAlg/FUSION /FusionAlg/BusToBusArray/BusToBusArray/FUS_Obj_38 ==
  <fus_output_38_obj> : Inport
  Bus Creator : BusCreator  Inputs=15  OutDataTypeStr=Bus: FUS_OBJ_TRACK_EST_ST  NonVirtualBus=on
      settings: InheritFromInputs=off
  Bus Creator1 : BusCreator  Inputs=15  OutDataTypeStr=Bus: FUS_OBJ_TRACK_PROP_ST  NonVirtualBus=on
      settings: InheritFromInputs=off
  Bus Creator2 : BusCreator  Inputs=10  OutDataTypeStr=Bus: FUS_OBJ_TRACK_INFO_ST  NonVirtualBus=on
      settings: InheritFromInputs=off
  Bus Creator3 : BusCreator  Inputs=3  OutDataTypeStr=Bus: FUS_OBJ_DATA_ST  NonVirtualBus=on
      settings: InheritFromInputs=off
  Bus Selector : BusSelector  OutputSignals=obj_estimate,obj_property,obj_information
  Bus Selector1 : BusSelector  OutputSignals=longPosition,latPosition,headingAngle,speed,yawRate,longRelativeVelocity,latRelativeVelocity,longAbsoluteVelocity,latAbsoluteVelocity,acceleration,longRelativeAcceleration,latRelativeAcceleration,longAbsoluteAcceleration,latAbsoluteAcceleration,curvature
  Bus Selector2 : BusSelector  OutputSignals=id,fusionSource,motionModel,trackStatus,positionConfidence,fcwConfidence,tjaConfidence,leftNearLaneMarkingConfidence,rightNearLaneMarkingConfidence,visionId,accelerationStdDev,headingAngleStdDev,latPositionStdDev,longPositionStdDev,speedStdDev
  Bus Selector3 : BusSelector  OutputSignals=valid,type,nearestSide,motionPatternCurrent,motionPatternHistory,width,height,length,distanceToleftNearLaneMarking,distanceToRightNearLaneMarking
  BUS_fus_output_38_obj : Outport
  wires:
  <fus_output_38_obj>/1 -> Bus Selector/1
  Bus Selector/1 -> Bus Selector1/1  "<obj_estimate>"
  Bus Selector1/1 -> Bus Creator/1  "<longPosition>"
  Bus Selector1/2 -> Bus Creator/2  "<latPosition>"
  Bus Selector1/4 -> Bus Creator/4  "<speed>"
  Bus Selector1/5 -> Bus Creator/5  "<yawRate>"
  Bus Selector1/6 -> Bus Creator/6  "<longRelativeVelocity>"
  Bus Selector1/3 -> Bus Creator/3  "<headingAngle>"
  Bus Selector1/7 -> Bus Creator/7  "<latRelativeVelocity>"
  Bus Selector/2 -> Bus Selector2/1  "<obj_property>"
  Bus Selector/3 -> Bus Selector3/1  "<obj_information>"
  Bus Selector2/1 -> Bus Creator1/1  "<id>"
  Bus Selector2/2 -> Bus Creator1/2  "<fusionSource>"
  Bus Selector2/3 -> Bus Creator1/3  "<motionModel>"
  Bus Selector2/4 -> Bus Creator1/4  "<trackStatus>"
  Bus Selector2/6 -> Bus Creator1/6  "<fcwConfidence>"
  Bus Selector2/11 -> Bus Creator1/11  "<accelerationStdDev>"
  Bus Selector2/12 -> Bus Creator1/12  "<headingAngleStdDev>"
  Bus Selector2/13 -> Bus Creator1/13  "<latPositionStdDev>"
  Bus Selector2/14 -> Bus Creator1/14  "<longPositionStdDev>"
  Bus Selector2/15 -> Bus Creator1/15  "<speedStdDev>"
  Bus Selector2/9 -> Bus Creator1/9  "<rightNearLaneMarkingConfidence>"
  Bus Selector2/8 -> Bus Creator1/8  "<leftNearLaneMarkingConfidence>"
  Bus Selector2/10 -> Bus Creator1/10  "<visionId>"
  Bus Selector2/5 -> Bus Creator1/5  "<positionConfidence>"
  Bus Selector2/7 -> Bus Creator1/7  "<tjaConfidence>"
  Bus Selector3/1 -> Bus Creator2/1  "<valid>"
  Bus Selector3/2 -> Bus Creator2/2  "<type>"
  Bus Selector3/3 -> Bus Creator2/3  "<nearestSide>"
  Bus Selector3/4 -> Bus Creator2/4  "<motionPatternCurrent>"
  Bus Selector3/5 -> Bus Creator2/5  "<motionPatternHistory>"
  Bus Selector3/6 -> Bus Creator2/6  "<width>"
  Bus Selector3/7 -> Bus Creator2/7  "<height>"
  Bus Selector3/8 -> Bus Creator2/8  "<length>"
  Bus Selector3/9 -> Bus Creator2/9  "<distanceToleftNearLaneMarking>"
  Bus Creator/1 -> Bus Creator3/1
  Bus Creator1/1 -> Bus Creator3/2
  Bus Creator2/1 -> Bus Creator3/3
  Bus Creator3/1 -> BUS_fus_output_38_obj/1
  Bus Selector3/10 -> Bus Creator2/10  "<distanceToRightNearLaneMarking>"
  Bus Selector1/8 -> Bus Creator/8  "<longAbsoluteVelocity>"
  Bus Selector1/9 -> Bus Creator/9  "<latAbsoluteVelocity>"
  Bus Selector1/10 -> Bus Creator/10  "<acceleration>"
  Bus Selector1/11 -> Bus Creator/11  "<longRelativeAcceleration>"
  Bus Selector1/12 -> Bus Creator/12  "<latRelativeAcceleration>"
  Bus Selector1/13 -> Bus Creator/13  "<longAbsoluteAcceleration>"
  Bus Selector1/14 -> Bus Creator/14  "<latAbsoluteAcceleration>"
  Bus Selector1/15 -> Bus Creator/15  "<curvature>"

== system fusionAlg/FUSION /FusionAlg/BusToBusArray/BusToBusArray/FUS_Obj_39 ==
  <fus_output_39_obj> : Inport
  Bus Creator : BusCreator  Inputs=15  OutDataTypeStr=Bus: FUS_OBJ_TRACK_EST_ST  NonVirtualBus=on
      settings: InheritFromInputs=off
  Bus Creator1 : BusCreator  Inputs=15  OutDataTypeStr=Bus: FUS_OBJ_TRACK_PROP_ST  NonVirtualBus=on
      settings: InheritFromInputs=off
  Bus Creator2 : BusCreator  Inputs=10  OutDataTypeStr=Bus: FUS_OBJ_TRACK_INFO_ST  NonVirtualBus=on
      settings: InheritFromInputs=off
  Bus Creator3 : BusCreator  Inputs=3  OutDataTypeStr=Bus: FUS_OBJ_DATA_ST  NonVirtualBus=on
      settings: InheritFromInputs=off
  Bus Selector : BusSelector  OutputSignals=obj_estimate,obj_property,obj_information
  Bus Selector1 : BusSelector  OutputSignals=longPosition,latPosition,headingAngle,speed,yawRate,longRelativeVelocity,latRelativeVelocity,longAbsoluteVelocity,latAbsoluteVelocity,acceleration,longRelativeAcceleration,latRelativeAcceleration,longAbsoluteAcceleration,latAbsoluteAcceleration,curvature
  Bus Selector2 : BusSelector  OutputSignals=id,fusionSource,motionModel,trackStatus,positionConfidence,fcwConfidence,tjaConfidence,leftNearLaneMarkingConfidence,rightNearLaneMarkingConfidence,visionId,accelerationStdDev,headingAngleStdDev,latPositionStdDev,longPositionStdDev,speedStdDev
  Bus Selector3 : BusSelector  OutputSignals=valid,type,nearestSide,motionPatternCurrent,motionPatternHistory,width,height,length,distanceToleftNearLaneMarking,distanceToRightNearLaneMarking
  BUS_fus_output_39_obj : Outport
  wires:
  <fus_output_39_obj>/1 -> Bus Selector/1
  Bus Selector/1 -> Bus Selector1/1  "<obj_estimate>"
  Bus Selector1/1 -> Bus Creator/1  "<longPosition>"
  Bus Selector1/2 -> Bus Creator/2  "<latPosition>"
  Bus Selector1/4 -> Bus Creator/4  "<speed>"
  Bus Selector1/5 -> Bus Creator/5  "<yawRate>"
  Bus Selector1/6 -> Bus Creator/6  "<longRelativeVelocity>"
  Bus Selector1/3 -> Bus Creator/3  "<headingAngle>"
  Bus Selector1/7 -> Bus Creator/7  "<latRelativeVelocity>"
  Bus Selector/2 -> Bus Selector2/1  "<obj_property>"
  Bus Selector/3 -> Bus Selector3/1  "<obj_information>"
  Bus Selector2/1 -> Bus Creator1/1  "<id>"
  Bus Selector2/2 -> Bus Creator1/2  "<fusionSource>"
  Bus Selector2/3 -> Bus Creator1/3  "<motionModel>"
  Bus Selector2/4 -> Bus Creator1/4  "<trackStatus>"
  Bus Selector2/6 -> Bus Creator1/6  "<fcwConfidence>"
  Bus Selector2/11 -> Bus Creator1/11  "<accelerationStdDev>"
  Bus Selector2/12 -> Bus Creator1/12  "<headingAngleStdDev>"
  Bus Selector2/13 -> Bus Creator1/13  "<latPositionStdDev>"
  Bus Selector2/14 -> Bus Creator1/14  "<longPositionStdDev>"
  Bus Selector2/15 -> Bus Creator1/15  "<speedStdDev>"
  Bus Selector2/9 -> Bus Creator1/9  "<rightNearLaneMarkingConfidence>"
  Bus Selector2/8 -> Bus Creator1/8  "<leftNearLaneMarkingConfidence>"
  Bus Selector2/10 -> Bus Creator1/10  "<visionId>"
  Bus Selector2/5 -> Bus Creator1/5  "<positionConfidence>"
  Bus Selector2/7 -> Bus Creator1/7  "<tjaConfidence>"
  Bus Selector3/1 -> Bus Creator2/1  "<valid>"
  Bus Selector3/2 -> Bus Creator2/2  "<type>"
  Bus Selector3/3 -> Bus Creator2/3  "<nearestSide>"
  Bus Selector3/4 -> Bus Creator2/4  "<motionPatternCurrent>"
  Bus Selector3/5 -> Bus Creator2/5  "<motionPatternHistory>"
  Bus Selector3/6 -> Bus Creator2/6  "<width>"
  Bus Selector3/7 -> Bus Creator2/7  "<height>"
  Bus Selector3/8 -> Bus Creator2/8  "<length>"
  Bus Selector3/9 -> Bus Creator2/9  "<distanceToleftNearLaneMarking>"
  Bus Creator/1 -> Bus Creator3/1
  Bus Creator1/1 -> Bus Creator3/2
  Bus Creator2/1 -> Bus Creator3/3
  Bus Creator3/1 -> BUS_fus_output_39_obj/1
  Bus Selector3/10 -> Bus Creator2/10  "<distanceToRightNearLaneMarking>"
  Bus Selector1/8 -> Bus Creator/8  "<longAbsoluteVelocity>"
  Bus Selector1/9 -> Bus Creator/9  "<latAbsoluteVelocity>"
  Bus Selector1/10 -> Bus Creator/10  "<acceleration>"
  Bus Selector1/11 -> Bus Creator/11  "<longRelativeAcceleration>"
  Bus Selector1/12 -> Bus Creator/12  "<latRelativeAcceleration>"
  Bus Selector1/13 -> Bus Creator/13  "<longAbsoluteAcceleration>"
  Bus Selector1/14 -> Bus Creator/14  "<latAbsoluteAcceleration>"
  Bus Selector1/15 -> Bus Creator/15  "<curvature>"

== system fusionAlg/FUSION /FusionAlg/BusToBusArray/BusToBusArray/FUS_Obj_4 ==
  <fus_output_04_obj> : Inport
  Bus Creator : BusCreator  Inputs=15  OutDataTypeStr=Bus: FUS_OBJ_TRACK_EST_ST  NonVirtualBus=on
      settings: InheritFromInputs=off
  Bus Creator1 : BusCreator  Inputs=15  OutDataTypeStr=Bus: FUS_OBJ_TRACK_PROP_ST  NonVirtualBus=on
      settings: InheritFromInputs=off
  Bus Creator2 : BusCreator  Inputs=10  OutDataTypeStr=Bus: FUS_OBJ_TRACK_INFO_ST  NonVirtualBus=on
      settings: InheritFromInputs=off
  Bus Creator3 : BusCreator  Inputs=3  OutDataTypeStr=Bus: FUS_OBJ_DATA_ST  NonVirtualBus=on
      settings: InheritFromInputs=off
  Bus Selector : BusSelector  OutputSignals=obj_estimate,obj_property,obj_information
  Bus Selector1 : BusSelector  OutputSignals=longPosition,latPosition,headingAngle,speed,yawRate,longRelativeVelocity,latRelativeVelocity,longAbsoluteVelocity,latAbsoluteVelocity,acceleration,longRelativeAcceleration,latRelativeAcceleration,longAbsoluteAcceleration,latAbsoluteAcceleration,curvature
  Bus Selector2 : BusSelector  OutputSignals=id,fusionSource,motionModel,trackStatus,positionConfidence,fcwConfidence,tjaConfidence,leftNearLaneMarkingConfidence,rightNearLaneMarkingConfidence,visionId,accelerationStdDev,headingAngleStdDev,latPositionStdDev,longPositionStdDev,speedStdDev
  Bus Selector3 : BusSelector  OutputSignals=valid,type,nearestSide,motionPatternCurrent,motionPatternHistory,width,height,length,distanceToleftNearLaneMarking,distanceToRightNearLaneMarking
  BUS_fus_output_04_obj : Outport
  wires:
  <fus_output_04_obj>/1 -> Bus Selector/1
  Bus Selector/1 -> Bus Selector1/1  "<obj_estimate>"
  Bus Selector1/1 -> Bus Creator/1  "<longPosition>"
  Bus Selector1/2 -> Bus Creator/2  "<latPosition>"
  Bus Selector1/4 -> Bus Creator/4  "<speed>"
  Bus Selector1/5 -> Bus Creator/5  "<yawRate>"
  Bus Selector1/6 -> Bus Creator/6  "<longRelativeVelocity>"
  Bus Selector1/3 -> Bus Creator/3  "<headingAngle>"
  Bus Selector1/7 -> Bus Creator/7  "<latRelativeVelocity>"
  Bus Selector/2 -> Bus Selector2/1  "<obj_property>"
  Bus Selector/3 -> Bus Selector3/1  "<obj_information>"
  Bus Selector2/1 -> Bus Creator1/1  "<id>"
  Bus Selector2/2 -> Bus Creator1/2  "<fusionSource>"
  Bus Selector2/3 -> Bus Creator1/3  "<motionModel>"
  Bus Selector2/4 -> Bus Creator1/4  "<trackStatus>"
  Bus Selector2/6 -> Bus Creator1/6  "<fcwConfidence>"
  Bus Selector2/11 -> Bus Creator1/11  "<accelerationStdDev>"
  Bus Selector2/12 -> Bus Creator1/12  "<headingAngleStdDev>"
  Bus Selector2/13 -> Bus Creator1/13  "<latPositionStdDev>"
  Bus Selector2/14 -> Bus Creator1/14  "<longPositionStdDev>"
  Bus Selector2/15 -> Bus Creator1/15  "<speedStdDev>"
  Bus Selector2/9 -> Bus Creator1/9  "<rightNearLaneMarkingConfidence>"
  Bus Selector2/8 -> Bus Creator1/8  "<leftNearLaneMarkingConfidence>"
  Bus Selector2/10 -> Bus Creator1/10  "<visionId>"
  Bus Selector2/5 -> Bus Creator1/5  "<positionConfidence>"
  Bus Selector2/7 -> Bus Creator1/7  "<tjaConfidence>"
  Bus Selector3/1 -> Bus Creator2/1  "<valid>"
  Bus Selector3/2 -> Bus Creator2/2  "<type>"
  Bus Selector3/3 -> Bus Creator2/3  "<nearestSide>"
  Bus Selector3/4 -> Bus Creator2/4  "<motionPatternCurrent>"
  Bus Selector3/5 -> Bus Creator2/5  "<motionPatternHistory>"
  Bus Selector3/6 -> Bus Creator2/6  "<width>"
  Bus Selector3/7 -> Bus Creator2/7  "<height>"
  Bus Selector3/8 -> Bus Creator2/8  "<length>"
  Bus Selector3/9 -> Bus Creator2/9  "<distanceToleftNearLaneMarking>"
  Bus Creator/1 -> Bus Creator3/1
  Bus Creator1/1 -> Bus Creator3/2
  Bus Creator2/1 -> Bus Creator3/3
  Bus Creator3/1 -> BUS_fus_output_04_obj/1
  Bus Selector3/10 -> Bus Creator2/10  "<distanceToRightNearLaneMarking>"
  Bus Selector1/8 -> Bus Creator/8  "<longAbsoluteVelocity>"
  Bus Selector1/9 -> Bus Creator/9  "<latAbsoluteVelocity>"
  Bus Selector1/10 -> Bus Creator/10  "<acceleration>"
  Bus Selector1/11 -> Bus Creator/11  "<longRelativeAcceleration>"
  Bus Selector1/12 -> Bus Creator/12  "<latRelativeAcceleration>"
  Bus Selector1/13 -> Bus Creator/13  "<longAbsoluteAcceleration>"
  Bus Selector1/14 -> Bus Creator/14  "<latAbsoluteAcceleration>"
  Bus Selector1/15 -> Bus Creator/15  "<curvature>"
